simulink library "xps_library"  (R2018a)
settings: Solver=ode45  StartTime=0.0  StopTime=10.0  RelTol=1e-3
undefined symbols (not defined in the file or in its folder): ip_name, lib_path
libraries: xbsIndex_r4 x2454, casper_library_flow_control x68, simulink x52, $bdroot x22, casper_library_misc x9
(part 5 of 27)

== system xps_library/ADCs/rfdc_V0_1 ==
  ch0_sim_a : Inport
  sim_sync : Inport  Port=2
  sim_ad_clk : Inport  Port=3
  ch0_delay_a{0..7} (8 alike) : Delay  DelayLength=1  InitialCondition=0  InputProcessing=Inherited
  ch0_downsample_a0 : DownSample  N=8  RateOptions=Allow multirate processing
  ch0_downsample_a1 : DownSample  N=8  phase=1  RateOptions=Allow multirate processing
  ch0_downsample_a2 : DownSample  N=8  phase=2  RateOptions=Allow multirate processing
  ch0_downsample_a3 : DownSample  N=8  phase=3  RateOptions=Allow multirate processing
  ch0_downsample_a4 : DownSample  N=8  phase=4  RateOptions=Allow multirate processing
  ch0_downsample_a5 : DownSample  N=8  phase=5  RateOptions=Allow multirate processing
  ch0_downsample_a6 : DownSample  N=8  phase=6  RateOptions=Allow multirate processing
  ch0_downsample_a7 : DownSample  N=8  phase=7  RateOptions=Allow multirate processing
  xps_library_ADCs_rfdc_V0_1_adc0_clk : xbsIndex_r4/Gateway In  gui_display_data_type=Boolean  arith_type=Boolean  n_bits=16  bin_pt=14  preci_type=Single  exp_width=8  frac_width=24  rows=1  columns=1  quantization="Round  (unbiased: +/- Inf)"  overflow=Saturate  period=1  UseAsADC=off  ADCChannel='1'  interface=None  automatic_assignment=on  address_offset=hex2dec('00')  intf_name=''  intf_description=''  default_value=0  timing_constraint=None  locs_specified=off  LOCs={}  io_standard={}  inherit_from_input=off  hdl_port=on  dbl_ovrd=off  block_type=gatewayin
  xps_library_ADCs_rfdc_V0_1_adc0_dout_{0..7} (8 alike) : xbsIndex_r4/Gateway In  gui_display_data_type=Fixed-point  arith_type=Unsigned  n_bits=16  bin_pt=0  preci_type=Single  exp_width=8  frac_width=24  rows=1  columns=1  quantization=Truncate  overflow=Wrap  period=1  UseAsADC=off  ADCChannel='1'  interface=None  automatic_assignment=on  address_offset=hex2dec('00')  intf_name=''  intf_description=''  default_value=0  timing_constraint=None  locs_specified=off  LOCs={}  io_standard={}  inherit_from_input=off  hdl_port=on  dbl_ovrd=off  block_type=gatewayin
  xps_library_ADCs_rfdc_V0_1_adc0_sync : xbsIndex_r4/Gateway In  gui_display_data_type=Boolean  arith_type=Boolean  n_bits=16  bin_pt=14  preci_type=Single  exp_width=8  frac_width=24  rows=1  columns=1  quantization="Round  (unbiased: +/- Inf)"  overflow=Saturate  period=1  UseAsADC=off  ADCChannel='1'  interface=None  automatic_assignment=on  address_offset=hex2dec('00')  intf_name=''  intf_description=''  default_value=0  timing_constraint=None  locs_specified=off  LOCs={}  io_standard={}  inherit_from_input=off  hdl_port=on  dbl_ovrd=off  block_type=gatewayin
  ch0_a0 : Outport
  ch0_a1 : Outport  Port=2
  ch0_a2 : Outport  Port=3
  ch0_a3 : Outport  Port=4
  ch0_a4 : Outport  Port=5
  ch0_a5 : Outport  Port=6
  ch0_a6 : Outport  Port=7
  ch0_a7 : Outport  Port=8
  sync_out : Outport  Port=9
  ad_clk_out : Outport  Port=10
  wires:
  ch0_sim_a/1 -> ch0_downsample_a2/1, ch0_downsample_a1/1, ch0_downsample_a3/1, ch0_downsample_a0/1, ch0_downsample_a4/1, ch0_downsample_a5/1, ch0_downsample_a6/1, ch0_downsample_a7/1
  ch0_downsample_a4/1 -> ch0_delay_a4/1
  ch0_downsample_a5/1 -> ch0_delay_a5/1
  ch0_downsample_a7/1 -> ch0_delay_a7/1
  xps_library_ADCs_rfdc_V0_1_adc0_dout_5/1 -> ch0_a5/1
  xps_library_ADCs_rfdc_V0_1_adc0_dout_4/1 -> ch0_a4/1
  ch0_delay_a4/1 -> xps_library_ADCs_rfdc_V0_1_adc0_dout_4/1
  xps_library_ADCs_rfdc_V0_1_adc0_dout_6/1 -> ch0_a6/1
  ch0_delay_a6/1 -> xps_library_ADCs_rfdc_V0_1_adc0_dout_6/1
  ch0_delay_a7/1 -> xps_library_ADCs_rfdc_V0_1_adc0_dout_7/1
  xps_library_ADCs_rfdc_V0_1_adc0_dout_7/1 -> ch0_a7/1
  ch0_downsample_a6/1 -> ch0_delay_a6/1
  ch0_delay_a5/1 -> xps_library_ADCs_rfdc_V0_1_adc0_dout_5/1
  xps_library_ADCs_rfdc_V0_1_adc0_clk/1 -> ad_clk_out/1
  sim_ad_clk/1 -> xps_library_ADCs_rfdc_V0_1_adc0_clk/1
  xps_library_ADCs_rfdc_V0_1_adc0_sync/1 -> sync_out/1
  sim_sync/1 -> xps_library_ADCs_rfdc_V0_1_adc0_sync/1
  xps_library_ADCs_rfdc_V0_1_adc0_dout_3/1 -> ch0_a3/1
  ch0_delay_a3/1 -> xps_library_ADCs_rfdc_V0_1_adc0_dout_3/1
  ch0_downsample_a3/1 -> ch0_delay_a3/1
  xps_library_ADCs_rfdc_V0_1_adc0_dout_2/1 -> ch0_a2/1
  ch0_delay_a2/1 -> xps_library_ADCs_rfdc_V0_1_adc0_dout_2/1
  ch0_downsample_a2/1 -> ch0_delay_a2/1
  xps_library_ADCs_rfdc_V0_1_adc0_dout_1/1 -> ch0_a1/1
  ch0_delay_a1/1 -> xps_library_ADCs_rfdc_V0_1_adc0_dout_1/1
  ch0_downsample_a1/1 -> ch0_delay_a1/1
  xps_library_ADCs_rfdc_V0_1_adc0_dout_0/1 -> ch0_a0/1
  ch0_delay_a0/1 -> xps_library_ADCs_rfdc_V0_1_adc0_dout_0/1
  ch0_downsample_a0/1 -> ch0_delay_a0/1

== system xps_library/ADCs/rfdc_V0_2 ==
  adc0_in_sim : Inport
  adc0_sync_in_sim : Inport  Port=2
  dac0_din : Inport  Port=3
  dac0_valid_in : Inport  Port=4
  Terminator : Terminator
  Terminator1 : Terminator
  rfdc_V0_2_rfdc_V0_2_adc0_dout : xbsIndex_r4/Gateway In  gui_display_data_type=Fixed-point  arith_type=Unsigned  n_bits=128  bin_pt=0  preci_type=Single  exp_width=8  frac_width=24  rows=1  columns=1  quantization=Truncate  overflow=Wrap  period=1  UseAsADC=off  ADCChannel='1'  interface=None  automatic_assignment=on  address_offset=hex2dec('00')  intf_name=''  intf_description=''  default_value=0  timing_constraint=None  locs_specified=off  LOCs={}  io_standard={}  inherit_from_input=off  hdl_port=on  dbl_ovrd=off  block_type=gatewayin
  rfdc_V0_2_rfdc_V0_2_adc0_sync : xbsIndex_r4/Gateway In  gui_display_data_type=Fixed-point  arith_type=Boolean  n_bits=1  bin_pt=0  preci_type=Single  exp_width=8  frac_width=24  rows=1  columns=1  quantization=Truncate  overflow=Wrap  period=1  UseAsADC=off  ADCChannel='1'  interface=None  automatic_assignment=on  address_offset=hex2dec('00')  intf_name=''  intf_description=''  default_value=0  timing_constraint=None  locs_specified=off  LOCs={}  io_standard={}  inherit_from_input=off  hdl_port=on  dbl_ovrd=off  block_type=gatewayin
  rfdc_V0_2_rfdc_V0_2_dac0_din : xbsIndex_r4/Gateway Out  inherit_from_input=off  hdl_port=on  rows=1  columns=1  UseAsDAC=off  DACChannel='1'  interface=None  automatic_assignment=on  address_offset=hex2dec('00')  intf_name=''  intf_description=''  timing_constraint=None  locs_specified=off  LOCs={}  io_standard={}  block_type=gatewayout
  rfdc_V0_2_rfdc_V0_2_dac0_valid : xbsIndex_r4/Gateway Out  inherit_from_input=off  hdl_port=on  rows=1  columns=1  UseAsDAC=off  DACChannel='1'  interface=None  automatic_assignment=on  address_offset=hex2dec('00')  intf_name=''  intf_description=''  timing_constraint=None  locs_specified=off  LOCs={}  io_standard={}  block_type=gatewayout
  adc0_dout : Outport
  adc0_sync_out : Outport  Port=2
  wires:
  rfdc_V0_2_rfdc_V0_2_dac0_valid/1 -> Terminator1/1
  dac0_valid_in/1 -> rfdc_V0_2_rfdc_V0_2_dac0_valid/1
  rfdc_V0_2_rfdc_V0_2_dac0_din/1 -> Terminator/1
  dac0_din/1 -> rfdc_V0_2_rfdc_V0_2_dac0_din/1
  rfdc_V0_2_rfdc_V0_2_adc0_sync/1 -> adc0_sync_out/1
  adc0_sync_in_sim/1 -> rfdc_V0_2_rfdc_V0_2_adc0_sync/1
  rfdc_V0_2_rfdc_V0_2_adc0_dout/1 -> adc0_dout/1
  adc0_in_sim/1 -> rfdc_V0_2_rfdc_V0_2_adc0_dout/1

== system xps_library/ADCs/rfdc_V0_3 ==
  adc0_in_sim : Inport
  adc0_sync_in_sim : Inport  Port=2
  rfdc_V0_3_rfdc_V0_3_adc0_dout : xbsIndex_r4/Gateway In  gui_display_data_type=Fixed-point  arith_type=Unsigned  n_bits=128  bin_pt=0  preci_type=Single  exp_width=8  frac_width=24  rows=1  columns=1  quantization=Truncate  overflow=Wrap  period=1  UseAsADC=off  ADCChannel='1'  interface=None  automatic_assignment=on  address_offset=hex2dec('00')  intf_name=''  intf_description=''  default_value=0  timing_constraint=None  locs_specified=off  LOCs={}  io_standard={}  inherit_from_input=off  hdl_port=on  dbl_ovrd=off  block_type=gatewayin
  rfdc_V0_3_rfdc_V0_3_adc0_sync : xbsIndex_r4/Gateway In  gui_display_data_type=Fixed-point  arith_type=Boolean  n_bits=1  bin_pt=0  preci_type=Single  exp_width=8  frac_width=24  rows=1  columns=1  quantization=Truncate  overflow=Wrap  period=1  UseAsADC=off  ADCChannel='1'  interface=None  automatic_assignment=on  address_offset=hex2dec('00')  intf_name=''  intf_description=''  default_value=0  timing_constraint=None  locs_specified=off  LOCs={}  io_standard={}  inherit_from_input=off  hdl_port=on  dbl_ovrd=off  block_type=gatewayin
  adc0_dout : Outport
  adc0_sync_out : Outport  Port=2
  wires:
  rfdc_V0_3_rfdc_V0_3_adc0_sync/1 -> adc0_sync_out/1
  adc0_sync_in_sim/1 -> rfdc_V0_3_rfdc_V0_3_adc0_sync/1
  rfdc_V0_3_rfdc_V0_3_adc0_dout/1 -> adc0_dout/1
  adc0_in_sim/1 -> rfdc_V0_3_rfdc_V0_3_adc0_dout/1

== system xps_library/ADCs/rfdc_V0_4 ==
  adc0_in_sim : Inport
  adc0_sync_in_sim : Inport  Port=2
  rfdc_V0_4_rfdc_V0_4_adc0_dout : xbsIndex_r4/Gateway In  gui_display_data_type=Fixed-point  arith_type=Unsigned  n_bits=128  bin_pt=0  preci_type=Single  exp_width=8  frac_width=24  rows=1  columns=1  quantization=Truncate  overflow=Wrap  period=1  UseAsADC=off  ADCChannel='1'  interface=None  automatic_assignment=on  address_offset=hex2dec('00')  intf_name=''  intf_description=''  default_value=0  timing_constraint=None  locs_specified=off  LOCs={}  io_standard={}  inherit_from_input=off  hdl_port=on  dbl_ovrd=off  block_type=gatewayin
  rfdc_V0_4_rfdc_V0_4_adc0_sync : xbsIndex_r4/Gateway In  gui_display_data_type=Fixed-point  arith_type=Boolean  n_bits=1  bin_pt=0  preci_type=Single  exp_width=8  frac_width=24  rows=1  columns=1  quantization=Truncate  overflow=Wrap  period=1  UseAsADC=off  ADCChannel='1'  interface=None  automatic_assignment=on  address_offset=hex2dec('00')  intf_name=''  intf_description=''  default_value=0  timing_constraint=None  locs_specified=off  LOCs={}  io_standard={}  inherit_from_input=off  hdl_port=on  dbl_ovrd=off  block_type=gatewayin
  adc0_dout : Outport
  adc0_sync_out : Outport  Port=2
  wires:
  rfdc_V0_4_rfdc_V0_4_adc0_sync/1 -> adc0_sync_out/1
  adc0_sync_in_sim/1 -> rfdc_V0_4_rfdc_V0_4_adc0_sync/1
  rfdc_V0_4_rfdc_V0_4_adc0_dout/1 -> adc0_dout/1
  adc0_in_sim/1 -> rfdc_V0_4_rfdc_V0_4_adc0_dout/1

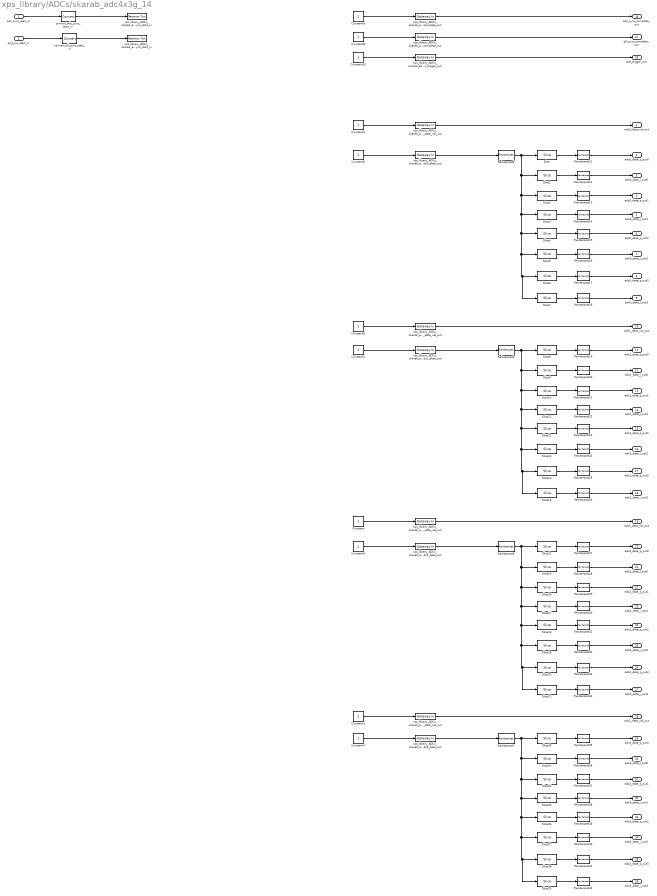
== system xps_library/ADCs/skarab_adc4x3g_14 ==
  adc_sync_start_in : Inport
  pll_sync_start_in : Inport  Port=2
  Constant{,1..10} (11 alike) : Constant
  Reinterpret{11..42} (32 alike) : xbsIndex_r4/Reinterpret  force_arith_type=on  arith_type="Signed  (2's comp)"  force_bin_pt=on  bin_pt=15  block_type=reinterpret
  Reinterpret{4..7} (4 alike) : xbsIndex_r4/Reinterpret  force_arith_type=on  arith_type=Unsigned  force_bin_pt=on  bin_pt=0  block_type=reinterpret
  Slice{,8,22,30} (4 alike) : xbsIndex_r4/Slice  nbits=16  boolean_output=off  mode=Lower Bit Location + Width  bit1=0  base1=MSB of Input  bit0=0  base0=LSB of Input  dbl_ovrd=off  block_type=slice
  Slice{1,9,23,31} (4 alike) : xbsIndex_r4/Slice  nbits=16  boolean_output=off  mode=Lower Bit Location + Width  bit1=0  base1=MSB of Input  bit0=16  base0=LSB of Input  dbl_ovrd=off  block_type=slice
  Slice{2,10,16,24} (4 alike) : xbsIndex_r4/Slice  nbits=16  boolean_output=off  mode=Lower Bit Location + Width  bit1=0  base1=MSB of Input  bit0=32  base0=LSB of Input  dbl_ovrd=off  block_type=slice
  Slice{3,11,17,25} (4 alike) : xbsIndex_r4/Slice  nbits=16  boolean_output=off  mode=Lower Bit Location + Width  bit1=0  base1=MSB of Input  bit0=48  base0=LSB of Input  dbl_ovrd=off  block_type=slice
  Slice{4,12,18,26} (4 alike) : xbsIndex_r4/Slice  nbits=16  boolean_output=off  mode=Lower Bit Location + Width  bit1=0  base1=MSB of Input  bit0=64  base0=LSB of Input  dbl_ovrd=off  block_type=slice
  Slice{5,13,19,27} (4 alike) : xbsIndex_r4/Slice  nbits=16  boolean_output=off  mode=Lower Bit Location + Width  bit1=0  base1=MSB of Input  bit0=80  base0=LSB of Input  dbl_ovrd=off  block_type=slice
  Slice{6,14,20,28} (4 alike) : xbsIndex_r4/Slice  nbits=16  boolean_output=off  mode=Lower Bit Location + Width  bit1=0  base1=MSB of Input  bit0=96  base0=LSB of Input  dbl_ovrd=off  block_type=slice
  Slice{7,15,21,29} (4 alike) : xbsIndex_r4/Slice  nbits=16  boolean_output=off  mode=Lower Bit Location + Width  bit1=0  base1=MSB of Input  bit0=112  base0=LSB of Input  dbl_ovrd=off  block_type=slice
  convert_adc_sync_start_in : xbsIndex_r4/Convert  gui_display_data_type=Boolean  arith_type=Boolean  n_bits=16  bin_pt=14  float_type=Single  exp_bits=8  fraction_bits=24  quantization=Truncate  overflow=Wrap  en=off  latency=0  pipeline=off  dbl_ovrd=off  block_type=convert
  convert_pll_sync_start_in : xbsIndex_r4/Convert  gui_display_data_type=Boolean  arith_type=Boolean  n_bits=16  bin_pt=14  float_type=Single  exp_bits=8  fraction_bits=24  quantization=Truncate  overflow=Wrap  en=off  latency=0  pipeline=off  dbl_ovrd=off  block_type=convert
  xps_library_ADCs_skarab_adc4x3g_14_adc0_data_out : xbsIndex_r4/Gateway In  gui_display_data_type=Fixed-point  arith_type=Unsigned  n_bits=128  bin_pt=0  preci_type=Single  exp_width=8  frac_width=24  rows=1  columns=1  quantization=Truncate  overflow=Wrap  period=1  UseAsADC=off  ADCChannel='1'  interface=None  automatic_assignment=on  address_offset=hex2dec('00')  intf_name=''  intf_description=''  default_value=0  timing_constraint=None  locs_specified=off  LOCs={}  io_standard={}  inherit_from_input=off  hdl_port=on  dbl_ovrd=off  block_type=gatewayin
  xps_library_ADCs_skarab_adc4x3g_14_adc0_data_val_out : xbsIndex_r4/Gateway In  gui_display_data_type=Boolean  arith_type=Boolean  n_bits=16  bin_pt=14  preci_type=Single  exp_width=8  frac_width=24  rows=1  columns=1  quantization="Round  (unbiased: +/- Inf)"  overflow=Saturate  period=1  UseAsADC=off  ADCChannel='1'  interface=None  automatic_assignment=on  address_offset=hex2dec('00')  intf_name=''  intf_description=''  default_value=0  timing_constraint=None  locs_specified=off  LOCs={}  io_standard={}  inherit_from_input=off  hdl_port=on  dbl_ovrd=off  block_type=gatewayin
  xps_library_ADCs_skarab_adc4x3g_14_adc1_data_out : xbsIndex_r4/Gateway In  gui_display_data_type=Fixed-point  arith_type=Unsigned  n_bits=128  bin_pt=0  preci_type=Single  exp_width=8  frac_width=24  rows=1  columns=1  quantization=Truncate  overflow=Wrap  period=1  UseAsADC=off  ADCChannel='1'  interface=None  automatic_assignment=on  address_offset=hex2dec('00')  intf_name=''  intf_description=''  default_value=0  timing_constraint=None  locs_specified=off  LOCs={}  io_standard={}  inherit_from_input=off  hdl_port=on  dbl_ovrd=off  block_type=gatewayin
  xps_library_ADCs_skarab_adc4x3g_14_adc1_data_val_out : xbsIndex_r4/Gateway In  gui_display_data_type=Boolean  arith_type=Boolean  n_bits=16  bin_pt=14  preci_type=Single  exp_width=8  frac_width=24  rows=1  columns=1  quantization="Round  (unbiased: +/- Inf)"  overflow=Saturate  period=1  UseAsADC=off  ADCChannel='1'  interface=None  automatic_assignment=on  address_offset=hex2dec('00')  intf_name=''  intf_description=''  default_value=0  timing_constraint=None  locs_specified=off  LOCs={}  io_standard={}  inherit_from_input=off  hdl_port=on  dbl_ovrd=off  block_type=gatewayin
  xps_library_ADCs_skarab_adc4x3g_14_adc2_data_out : xbsIndex_r4/Gateway In  gui_display_data_type=Fixed-point  arith_type=Unsigned  n_bits=128  bin_pt=0  preci_type=Single  exp_width=8  frac_width=24  rows=1  columns=1  quantization=Truncate  overflow=Wrap  period=1  UseAsADC=off  ADCChannel='1'  interface=None  automatic_assignment=on  address_offset=hex2dec('00')  intf_name=''  intf_description=''  default_value=0  timing_constraint=None  locs_specified=off  LOCs={}  io_standard={}  inherit_from_input=off  hdl_port=on  dbl_ovrd=off  block_type=gatewayin
  xps_library_ADCs_skarab_adc4x3g_14_adc2_data_val_out : xbsIndex_r4/Gateway In  gui_display_data_type=Boolean  arith_type=Boolean  n_bits=16  bin_pt=14  preci_type=Single  exp_width=8  frac_width=24  rows=1  columns=1  quantization="Round  (unbiased: +/- Inf)"  overflow=Saturate  period=1  UseAsADC=off  ADCChannel='1'  interface=None  automatic_assignment=on  address_offset=hex2dec('00')  intf_name=''  intf_description=''  default_value=0  timing_constraint=None  locs_specified=off  LOCs={}  io_standard={}  inherit_from_input=off  hdl_port=on  dbl_ovrd=off  block_type=gatewayin
  xps_library_ADCs_skarab_adc4x3g_14_adc3_data_out : xbsIndex_r4/Gateway In  gui_display_data_type=Fixed-point  arith_type=Unsigned  n_bits=128  bin_pt=0  preci_type=Single  exp_width=8  frac_width=24  rows=1  columns=1  quantization=Truncate  overflow=Wrap  period=1  UseAsADC=off  ADCChannel='1'  interface=None  automatic_assignment=on  address_offset=hex2dec('00')  intf_name=''  intf_description=''  default_value=0  timing_constraint=None  locs_specified=off  LOCs={}  io_standard={}  inherit_from_input=off  hdl_port=on  dbl_ovrd=off  block_type=gatewayin
  xps_library_ADCs_skarab_adc4x3g_14_adc3_data_val_out : xbsIndex_r4/Gateway In  gui_display_data_type=Boolean  arith_type=Boolean  n_bits=16  bin_pt=14  preci_type=Single  exp_width=8  frac_width=24  rows=1  columns=1  quantization="Round  (unbiased: +/- Inf)"  overflow=Saturate  period=1  UseAsADC=off  ADCChannel='1'  interface=None  automatic_assignment=on  address_offset=hex2dec('00')  intf_name=''  intf_description=''  default_value=0  timing_constraint=None  locs_specified=off  LOCs={}  io_standard={}  inherit_from_input=off  hdl_port=on  dbl_ovrd=off  block_type=gatewayin
  xps_library_ADCs_skarab_adc4x3g_14_adc_sync_complete_out : xbsIndex_r4/Gateway In  gui_display_data_type=Boolean  arith_type=Boolean  n_bits=16  bin_pt=14  preci_type=Single  exp_width=8  frac_width=24  rows=1  columns=1  quantization="Round  (unbiased: +/- Inf)"  overflow=Saturate  period=1  UseAsADC=off  ADCChannel='1'  interface=None  automatic_assignment=on  address_offset=hex2dec('00')  intf_name=''  intf_description=''  default_value=0  timing_constraint=None  locs_specified=off  LOCs={}  io_standard={}  inherit_from_input=off  hdl_port=on  dbl_ovrd=off  block_type=gatewayin
  xps_library_ADCs_skarab_adc4x3g_14_adc_sync_start_in : xbsIndex_r4/Gateway Out  inherit_from_input=off  hdl_port=on  rows=1  columns=1  UseAsDAC=off  DACChannel='1'  interface=None  automatic_assignment=on  address_offset=hex2dec('00')  intf_name=''  intf_description=''  timing_constraint=None  locs_specified=off  LOCs={}  io_standard={}  block_type=gatewayout
  xps_library_ADCs_skarab_adc4x3g_14_adc_trigger_out : xbsIndex_r4/Gateway In  gui_display_data_type=Boolean  arith_type=Boolean  n_bits=16  bin_pt=14  preci_type=Single  exp_width=8  frac_width=24  rows=1  columns=1  quantization="Round  (unbiased: +/- Inf)"  overflow=Saturate  period=1  UseAsADC=off  ADCChannel='1'  interface=None  automatic_assignment=on  address_offset=hex2dec('00')  intf_name=''  intf_description=''  default_value=0  timing_constraint=None  locs_specified=off  LOCs={}  io_standard={}  inherit_from_input=off  hdl_port=on  dbl_ovrd=off  block_type=gatewayin
  xps_library_ADCs_skarab_adc4x3g_14_pll_sync_complete_out : xbsIndex_r4/Gateway In  gui_display_data_type=Boolean  arith_type=Boolean  n_bits=16  bin_pt=14  preci_type=Single  exp_width=8  frac_width=24  rows=1  columns=1  quantization="Round  (unbiased: +/- Inf)"  overflow=Saturate  period=1  UseAsADC=off  ADCChannel='1'  interface=None  automatic_assignment=on  address_offset=hex2dec('00')  intf_name=''  intf_description=''  default_value=0  timing_constraint=None  locs_specified=off  LOCs={}  io_standard={}  inherit_from_input=off  hdl_port=on  dbl_ovrd=off  block_type=gatewayin
  xps_library_ADCs_skarab_adc4x3g_14_pll_sync_start_in : xbsIndex_r4/Gateway Out  inherit_from_input=off  hdl_port=on  rows=1  columns=1  UseAsDAC=off  DACChannel='1'  interface=None  automatic_assignment=on  address_offset=hex2dec('00')  intf_name=''  intf_description=''  timing_constraint=None  locs_specified=off  LOCs={}  io_standard={}  block_type=gatewayout
  adc0_data_val_out : Outport
  adc0_data_q_out0 : Outport  Port=2
  adc0_data_i_out0 : Outport  Port=3
  adc0_data_q_out1 : Outport  Port=4
  adc0_data_i_out1 : Outport  Port=5
  adc0_data_q_out2 : Outport  Port=6
  adc0_data_i_out2 : Outport  Port=7
  adc0_data_q_out3 : Outport  Port=8
  adc0_data_i_out3 : Outport  Port=9
  adc1_data_val_out : Outport  Port=10
  adc1_data_q_out0 : Outport  Port=11
  adc1_data_i_out0 : Outport  Port=12
  adc1_data_q_out1 : Outport  Port=13
  adc1_data_i_out1 : Outport  Port=14
  adc1_data_q_out2 : Outport  Port=15
  adc1_data_i_out2 : Outport  Port=16
  adc1_data_q_out3 : Outport  Port=17
  adc1_data_i_out3 : Outport  Port=18
  adc2_data_val_out : Outport  Port=19
  adc2_data_q_out0 : Outport  Port=20
  adc2_data_i_out0 : Outport  Port=21
  adc2_data_q_out1 : Outport  Port=22
  adc2_data_i_out1 : Outport  Port=23
  adc2_data_q_out2 : Outport  Port=24
  adc2_data_i_out2 : Outport  Port=25
  adc2_data_q_out3 : Outport  Port=26
  adc2_data_i_out3 : Outport  Port=27
  adc3_data_val_out : Outport  Port=28
  adc3_data_q_out0 : Outport  Port=29
  adc3_data_i_out0 : Outport  Port=30
  adc3_data_q_out1 : Outport  Port=31
  adc3_data_i_out1 : Outport  Port=32
  adc3_data_q_out2 : Outport  Port=33
  adc3_data_i_out2 : Outport  Port=34
  adc3_data_q_out3 : Outport  Port=35
  adc3_data_i_out3 : Outport  Port=36
  pll_sync_complete_out : Outport  Port=37
  adc_sync_complete_out : Outport  Port=38
  adc_trigger_out : Outport  Port=39
  wires:
  xps_library_ADCs_skarab_adc4x3g_14_adc_trigger_out/1 -> adc_trigger_out/1
  Constant10/1 -> xps_library_ADCs_skarab_adc4x3g_14_adc_trigger_out/1
  xps_library_ADCs_skarab_adc4x3g_14_adc_sync_complete_out/1 -> adc_sync_complete_out/1
  Constant9/1 -> xps_library_ADCs_skarab_adc4x3g_14_adc_sync_complete_out/1
  xps_library_ADCs_skarab_adc4x3g_14_pll_sync_complete_out/1 -> pll_sync_complete_out/1
  Constant8/1 -> xps_library_ADCs_skarab_adc4x3g_14_pll_sync_complete_out/1
  Slice29/1 -> Reinterpret42/1
  Reinterpret42/1 -> adc3_data_i_out3/1
  Slice28/1 -> Reinterpret41/1
  Reinterpret41/1 -> adc3_data_q_out3/1
  Slice27/1 -> Reinterpret40/1
  Reinterpret40/1 -> adc3_data_i_out2/1
  Slice26/1 -> Reinterpret39/1
  Reinterpret39/1 -> adc3_data_q_out2/1
  Slice25/1 -> Reinterpret38/1
  Reinterpret38/1 -> adc3_data_i_out1/1
  Slice24/1 -> Reinterpret37/1
  Reinterpret37/1 -> adc3_data_q_out1/1
  Slice31/1 -> Reinterpret36/1
  Reinterpret36/1 -> adc3_data_i_out0/1
  Slice30/1 -> Reinterpret35/1
  Reinterpret35/1 -> adc3_data_q_out0/1
  Reinterpret7/1 -> Slice30/1, Slice31/1, Slice24/1, Slice25/1, Slice26/1, Slice27/1, Slice28/1, Slice29/1
  xps_library_ADCs_skarab_adc4x3g_14_adc3_data_out/1 -> Reinterpret7/1
  Constant7/1 -> xps_library_ADCs_skarab_adc4x3g_14_adc3_data_out/1
  Slice21/1 -> Reinterpret34/1
  Reinterpret34/1 -> adc2_data_i_out3/1
  Slice20/1 -> Reinterpret33/1
  Reinterpret33/1 -> adc2_data_q_out3/1
  Slice19/1 -> Reinterpret32/1
  Reinterpret32/1 -> adc2_data_i_out2/1
  Slice18/1 -> Reinterpret31/1
  Reinterpret31/1 -> adc2_data_q_out2/1
  Slice17/1 -> Reinterpret30/1
  Reinterpret30/1 -> adc2_data_i_out1/1
  Slice16/1 -> Reinterpret29/1
  Reinterpret29/1 -> adc2_data_q_out1/1
  Slice23/1 -> Reinterpret28/1
  Reinterpret28/1 -> adc2_data_i_out0/1
  Slice22/1 -> Reinterpret27/1
  Reinterpret27/1 -> adc2_data_q_out0/1
  Reinterpret5/1 -> Slice22/1, Slice23/1, Slice16/1, Slice17/1, Slice18/1, Slice19/1, Slice20/1, Slice21/1
  xps_library_ADCs_skarab_adc4x3g_14_adc2_data_out/1 -> Reinterpret5/1
  Constant3/1 -> xps_library_ADCs_skarab_adc4x3g_14_adc2_data_out/1
  Slice15/1 -> Reinterpret26/1
  Reinterpret26/1 -> adc1_data_i_out3/1
  Slice14/1 -> Reinterpret25/1
  Reinterpret25/1 -> adc1_data_q_out3/1
  Slice13/1 -> Reinterpret24/1
  Reinterpret24/1 -> adc1_data_i_out2/1
  Slice12/1 -> Reinterpret23/1
  Reinterpret23/1 -> adc1_data_q_out2/1
  Slice11/1 -> Reinterpret22/1
  Reinterpret22/1 -> adc1_data_i_out1/1
  Slice10/1 -> Reinterpret21/1
  Reinterpret21/1 -> adc1_data_q_out1/1
  Slice9/1 -> Reinterpret20/1
  Reinterpret20/1 -> adc1_data_i_out0/1
  Slice8/1 -> Reinterpret19/1
  Reinterpret19/1 -> adc1_data_q_out0/1
  Reinterpret4/1 -> Slice8/1, Slice9/1, Slice10/1, Slice11/1, Slice12/1, Slice13/1, Slice14/1, Slice15/1
  xps_library_ADCs_skarab_adc4x3g_14_adc1_data_out/1 -> Reinterpret4/1
  Constant2/1 -> xps_library_ADCs_skarab_adc4x3g_14_adc1_data_out/1
  Slice7/1 -> Reinterpret18/1
  Reinterpret18/1 -> adc0_data_i_out3/1
  Slice6/1 -> Reinterpret17/1
  Reinterpret17/1 -> adc0_data_q_out3/1
  Slice5/1 -> Reinterpret16/1
  Reinterpret16/1 -> adc0_data_i_out2/1
  Slice4/1 -> Reinterpret15/1
  Reinterpret15/1 -> adc0_data_q_out2/1
  Slice3/1 -> Reinterpret14/1
  Reinterpret14/1 -> adc0_data_i_out1/1
  Slice2/1 -> Reinterpret13/1
  Reinterpret13/1 -> adc0_data_q_out1/1
  Slice1/1 -> Reinterpret12/1
  Reinterpret12/1 -> adc0_data_i_out0/1
  Slice/1 -> Reinterpret11/1
  Reinterpret11/1 -> adc0_data_q_out0/1
  Reinterpret6/1 -> Slice/1, Slice1/1, Slice2/1, Slice3/1, Slice4/1, Slice5/1, Slice6/1, Slice7/1
  xps_library_ADCs_skarab_adc4x3g_14_adc0_data_out/1 -> Reinterpret6/1
  Constant6/1 -> xps_library_ADCs_skarab_adc4x3g_14_adc0_data_out/1
  xps_library_ADCs_skarab_adc4x3g_14_adc1_data_val_out/1 -> adc1_data_val_out/1
  Constant5/1 -> xps_library_ADCs_skarab_adc4x3g_14_adc1_data_val_out/1
  xps_library_ADCs_skarab_adc4x3g_14_adc0_data_val_out/1 -> adc0_data_val_out/1
  Constant4/1 -> xps_library_ADCs_skarab_adc4x3g_14_adc0_data_val_out/1
  xps_library_ADCs_skarab_adc4x3g_14_adc3_data_val_out/1 -> adc3_data_val_out/1
  Constant1/1 -> xps_library_ADCs_skarab_adc4x3g_14_adc3_data_val_out/1
  xps_library_ADCs_skarab_adc4x3g_14_adc2_data_val_out/1 -> adc2_data_val_out/1
  Constant/1 -> xps_library_ADCs_skarab_adc4x3g_14_adc2_data_val_out/1
  convert_pll_sync_start_in/1 -> xps_library_ADCs_skarab_adc4x3g_14_pll_sync_start_in/1
  pll_sync_start_in/1 -> convert_pll_sync_start_in/1
  convert_adc_sync_start_in/1 -> xps_library_ADCs_skarab_adc4x3g_14_adc_sync_start_in/1
  adc_sync_start_in/1 -> convert_adc_sync_start_in/1

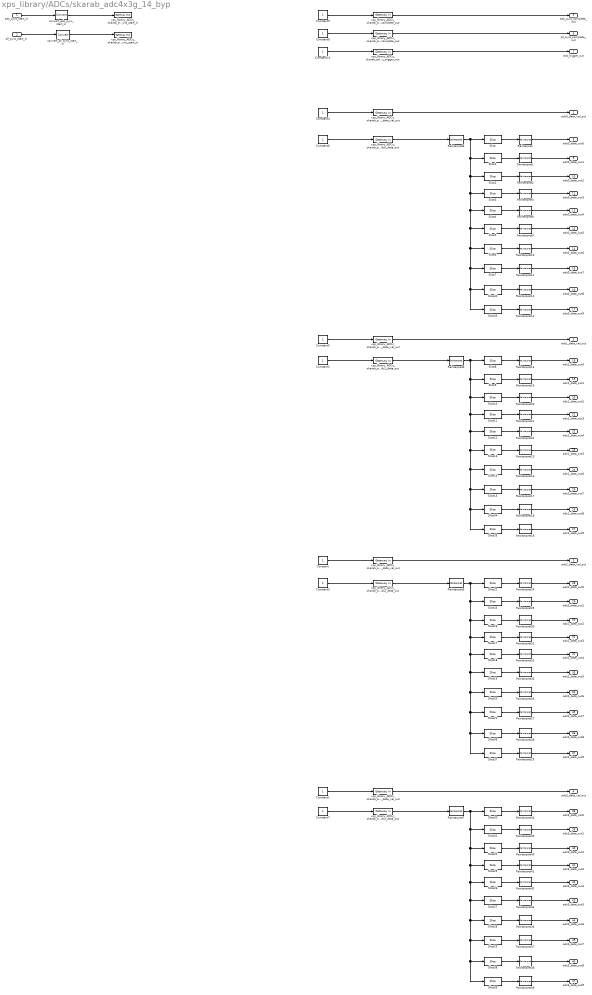
== system xps_library/ADCs/skarab_adc4x3g_14_byp ==
  adc_sync_start_in : Inport
  pll_sync_start_in : Inport  Port=2
  Constant{,1..10} (11 alike) : Constant
  Reinterpret{,1..3,8..43} (40 alike) : xbsIndex_r4/Reinterpret  force_arith_type=on  arith_type="Signed  (2's comp)"  force_bin_pt=on  bin_pt=11  block_type=reinterpret
  Reinterpret{4..7} (4 alike) : xbsIndex_r4/Reinterpret  force_arith_type=on  arith_type=Unsigned  force_bin_pt=on  bin_pt=0  block_type=reinterpret
  Slice{,8,22,30} (4 alike) : xbsIndex_r4/Slice  nbits=12  boolean_output=off  mode=Lower Bit Location + Width  bit1=0  base1=MSB of Input  bit0=0  base0=LSB of Input  dbl_ovrd=off  block_type=slice
  Slice{1,9,23,31} (4 alike) : xbsIndex_r4/Slice  nbits=12  boolean_output=off  mode=Lower Bit Location + Width  bit1=0  base1=MSB of Input  bit0=12  base0=LSB of Input  dbl_ovrd=off  block_type=slice
  Slice{2,10,16,24} (4 alike) : xbsIndex_r4/Slice  nbits=12  boolean_output=off  mode=Lower Bit Location + Width  bit1=0  base1=MSB of Input  bit0=24  base0=LSB of Input  dbl_ovrd=off  block_type=slice
  Slice{3,11,17,25} (4 alike) : xbsIndex_r4/Slice  nbits=12  boolean_output=off  mode=Lower Bit Location + Width  bit1=0  base1=MSB of Input  bit0=36  base0=LSB of Input  dbl_ovrd=off  block_type=slice
  Slice{4,12,18,26} (4 alike) : xbsIndex_r4/Slice  nbits=12  boolean_output=off  mode=Lower Bit Location + Width  bit1=0  base1=MSB of Input  bit0=48  base0=LSB of Input  dbl_ovrd=off  block_type=slice
  Slice{5,13,19,27} (4 alike) : xbsIndex_r4/Slice  nbits=12  boolean_output=off  mode=Lower Bit Location + Width  bit1=0  base1=MSB of Input  bit0=60  base0=LSB of Input  dbl_ovrd=off  block_type=slice
  Slice{6,14,20,28} (4 alike) : xbsIndex_r4/Slice  nbits=12  boolean_output=off  mode=Lower Bit Location + Width  bit1=0  base1=MSB of Input  bit0=72  base0=LSB of Input  dbl_ovrd=off  block_type=slice
  Slice{7,15,21,29} (4 alike) : xbsIndex_r4/Slice  nbits=12  boolean_output=off  mode=Lower Bit Location + Width  bit1=0  base1=MSB of Input  bit0=84  base0=LSB of Input  dbl_ovrd=off  block_type=slice
  Slice{32,34,36,38} (4 alike) : xbsIndex_r4/Slice  nbits=12  boolean_output=off  mode=Lower Bit Location + Width  bit1=0  base1=MSB of Input  bit0=96  base0=LSB of Input  dbl_ovrd=off  block_type=slice
  Slice{33,35,37,39} (4 alike) : xbsIndex_r4/Slice  nbits=12  boolean_output=off  mode=Lower Bit Location + Width  bit1=0  base1=MSB of Input  bit0=108  base0=LSB of Input  dbl_ovrd=off  block_type=slice
  convert_adc_sync_start_in : xbsIndex_r4/Convert  gui_display_data_type=Boolean  arith_type=Boolean  n_bits=16  bin_pt=14  float_type=Single  exp_bits=8  fraction_bits=24  quantization=Truncate  overflow=Wrap  en=off  latency=0  pipeline=off  dbl_ovrd=off  block_type=convert
  convert_pll_sync_start_in : xbsIndex_r4/Convert  gui_display_data_type=Boolean  arith_type=Boolean  n_bits=16  bin_pt=14  float_type=Single  exp_bits=8  fraction_bits=24  quantization=Truncate  overflow=Wrap  en=off  latency=0  pipeline=off  dbl_ovrd=off  block_type=convert
  xps_library_ADCs_skarab_adc4x3g_14_byp_adc0_data_out : xbsIndex_r4/Gateway In  gui_display_data_type=Fixed-point  arith_type=Unsigned  n_bits=128  bin_pt=0  preci_type=Single  exp_width=8  frac_width=24  rows=1  columns=1  quantization=Truncate  overflow=Wrap  period=1  UseAsADC=off  ADCChannel='1'  interface=None  automatic_assignment=on  address_offset=hex2dec('00')  intf_name=''  intf_description=''  default_value=0  timing_constraint=None  locs_specified=off  LOCs={}  io_standard={}  inherit_from_input=off  hdl_port=on  dbl_ovrd=off  block_type=gatewayin
  xps_library_ADCs_skarab_adc4x3g_14_byp_adc0_data_val_out : xbsIndex_r4/Gateway In  gui_display_data_type=Boolean  arith_type=Boolean  n_bits=16  bin_pt=14  preci_type=Single  exp_width=8  frac_width=24  rows=1  columns=1  quantization="Round  (unbiased: +/- Inf)"  overflow=Saturate  period=1  UseAsADC=off  ADCChannel='1'  interface=None  automatic_assignment=on  address_offset=hex2dec('00')  intf_name=''  intf_description=''  default_value=0  timing_constraint=None  locs_specified=off  LOCs={}  io_standard={}  inherit_from_input=off  hdl_port=on  dbl_ovrd=off  block_type=gatewayin
  xps_library_ADCs_skarab_adc4x3g_14_byp_adc1_data_out : xbsIndex_r4/Gateway In  gui_display_data_type=Fixed-point  arith_type=Unsigned  n_bits=128  bin_pt=0  preci_type=Single  exp_width=8  frac_width=24  rows=1  columns=1  quantization=Truncate  overflow=Wrap  period=1  UseAsADC=off  ADCChannel='1'  interface=None  automatic_assignment=on  address_offset=hex2dec('00')  intf_name=''  intf_description=''  default_value=0  timing_constraint=None  locs_specified=off  LOCs={}  io_standard={}  inherit_from_input=off  hdl_port=on  dbl_ovrd=off  block_type=gatewayin
  xps_library_ADCs_skarab_adc4x3g_14_byp_adc1_data_val_out : xbsIndex_r4/Gateway In  gui_display_data_type=Boolean  arith_type=Boolean  n_bits=16  bin_pt=14  preci_type=Single  exp_width=8  frac_width=24  rows=1  columns=1  quantization="Round  (unbiased: +/- Inf)"  overflow=Saturate  period=1  UseAsADC=off  ADCChannel='1'  interface=None  automatic_assignment=on  address_offset=hex2dec('00')  intf_name=''  intf_description=''  default_value=0  timing_constraint=None  locs_specified=off  LOCs={}  io_standard={}  inherit_from_input=off  hdl_port=on  dbl_ovrd=off  block_type=gatewayin
  xps_library_ADCs_skarab_adc4x3g_14_byp_adc2_data_out : xbsIndex_r4/Gateway In  gui_display_data_type=Fixed-point  arith_type=Unsigned  n_bits=128  bin_pt=0  preci_type=Single  exp_width=8  frac_width=24  rows=1  columns=1  quantization=Truncate  overflow=Wrap  period=1  UseAsADC=off  ADCChannel='1'  interface=None  automatic_assignment=on  address_offset=hex2dec('00')  intf_name=''  intf_description=''  default_value=0  timing_constraint=None  locs_specified=off  LOCs={}  io_standard={}  inherit_from_input=off  hdl_port=on  dbl_ovrd=off  block_type=gatewayin
  xps_library_ADCs_skarab_adc4x3g_14_byp_adc2_data_val_out : xbsIndex_r4/Gateway In  gui_display_data_type=Boolean  arith_type=Boolean  n_bits=16  bin_pt=14  preci_type=Single  exp_width=8  frac_width=24  rows=1  columns=1  quantization="Round  (unbiased: +/- Inf)"  overflow=Saturate  period=1  UseAsADC=off  ADCChannel='1'  interface=None  automatic_assignment=on  address_offset=hex2dec('00')  intf_name=''  intf_description=''  default_value=0  timing_constraint=None  locs_specified=off  LOCs={}  io_standard={}  inherit_from_input=off  hdl_port=on  dbl_ovrd=off  block_type=gatewayin
  xps_library_ADCs_skarab_adc4x3g_14_byp_adc3_data_out : xbsIndex_r4/Gateway In  gui_display_data_type=Fixed-point  arith_type=Unsigned  n_bits=128  bin_pt=0  preci_type=Single  exp_width=8  frac_width=24  rows=1  columns=1  quantization=Truncate  overflow=Wrap  period=1  UseAsADC=off  ADCChannel='1'  interface=None  automatic_assignment=on  address_offset=hex2dec('00')  intf_name=''  intf_description=''  default_value=0  timing_constraint=None  locs_specified=off  LOCs={}  io_standard={}  inherit_from_input=off  hdl_port=on  dbl_ovrd=off  block_type=gatewayin
  xps_library_ADCs_skarab_adc4x3g_14_byp_adc3_data_val_out : xbsIndex_r4/Gateway In  gui_display_data_type=Boolean  arith_type=Boolean  n_bits=16  bin_pt=14  preci_type=Single  exp_width=8  frac_width=24  rows=1  columns=1  quantization="Round  (unbiased: +/- Inf)"  overflow=Saturate  period=1  UseAsADC=off  ADCChannel='1'  interface=None  automatic_assignment=on  address_offset=hex2dec('00')  intf_name=''  intf_description=''  default_value=0  timing_constraint=None  locs_specified=off  LOCs={}  io_standard={}  inherit_from_input=off  hdl_port=on  dbl_ovrd=off  block_type=gatewayin
  xps_library_ADCs_skarab_adc4x3g_14_byp_adc_sync_complete_out : xbsIndex_r4/Gateway In  gui_display_data_type=Boolean  arith_type=Boolean  n_bits=16  bin_pt=14  preci_type=Single  exp_width=8  frac_width=24  rows=1  columns=1  quantization="Round  (unbiased: +/- Inf)"  overflow=Saturate  period=1  UseAsADC=off  ADCChannel='1'  interface=None  automatic_assignment=on  address_offset=hex2dec('00')  intf_name=''  intf_description=''  default_value=0  timing_constraint=None  locs_specified=off  LOCs={}  io_standard={}  inherit_from_input=off  hdl_port=on  dbl_ovrd=off  block_type=gatewayin
  xps_library_ADCs_skarab_adc4x3g_14_byp_adc_sync_start_in : xbsIndex_r4/Gateway Out  inherit_from_input=off  hdl_port=on  rows=1  columns=1  UseAsDAC=off  DACChannel='1'  interface=None  automatic_assignment=on  address_offset=hex2dec('00')  intf_name=''  intf_description=''  timing_constraint=None  locs_specified=off  LOCs={}  io_standard={}  block_type=gatewayout
  xps_library_ADCs_skarab_adc4x3g_14_byp_adc_trigger_out : xbsIndex_r4/Gateway In  gui_display_data_type=Boolean  arith_type=Boolean  n_bits=16  bin_pt=14  preci_type=Single  exp_width=8  frac_width=24  rows=1  columns=1  quantization="Round  (unbiased: +/- Inf)"  overflow=Saturate  period=1  UseAsADC=off  ADCChannel='1'  interface=None  automatic_assignment=on  address_offset=hex2dec('00')  intf_name=''  intf_description=''  default_value=0  timing_constraint=None  locs_specified=off  LOCs={}  io_standard={}  inherit_from_input=off  hdl_port=on  dbl_ovrd=off  block_type=gatewayin
  xps_library_ADCs_skarab_adc4x3g_14_byp_pll_sync_complete_out : xbsIndex_r4/Gateway In  gui_display_data_type=Boolean  arith_type=Boolean  n_bits=16  bin_pt=14  preci_type=Single  exp_width=8  frac_width=24  rows=1  columns=1  quantization="Round  (unbiased: +/- Inf)"  overflow=Saturate  period=1  UseAsADC=off  ADCChannel='1'  interface=None  automatic_assignment=on  address_offset=hex2dec('00')  intf_name=''  intf_description=''  default_value=0  timing_constraint=None  locs_specified=off  LOCs={}  io_standard={}  inherit_from_input=off  hdl_port=on  dbl_ovrd=off  block_type=gatewayin
  xps_library_ADCs_skarab_adc4x3g_14_byp_pll_sync_start_in : xbsIndex_r4/Gateway Out  inherit_from_input=off  hdl_port=on  rows=1  columns=1  UseAsDAC=off  DACChannel='1'  interface=None  automatic_assignment=on  address_offset=hex2dec('00')  intf_name=''  intf_description=''  timing_constraint=None  locs_specified=off  LOCs={}  io_standard={}  block_type=gatewayout
  adc0_data_val_out : Outport
  adc1_data_val_out : Outport  Port=2
  adc2_data_val_out : Outport  Port=3
  adc3_data_val_out : Outport  Port=4
  pll_sync_complete_out : Outport  Port=5
  adc_sync_complete_out : Outport  Port=6
  adc_trigger_out : Outport  Port=7
  adc0_data_out0 : Outport  Port=8
  adc0_data_out1 : Outport  Port=9
  adc0_data_out2 : Outport  Port=10
  adc0_data_out3 : Outport  Port=11
  adc0_data_out4 : Outport  Port=12
  adc0_data_out5 : Outport  Port=13
  adc0_data_out6 : Outport  Port=14
  adc0_data_out7 : Outport  Port=15
  adc0_data_out8 : Outport  Port=16
  adc0_data_out9 : Outport  Port=17
  adc1_data_out0 : Outport  Port=18
  adc1_data_out1 : Outport  Port=19
  adc1_data_out2 : Outport  Port=20
  adc1_data_out3 : Outport  Port=21
  adc1_data_out4 : Outport  Port=22
  adc1_data_out5 : Outport  Port=23
  adc1_data_out6 : Outport  Port=24
  adc1_data_out7 : Outport  Port=25
  adc1_data_out8 : Outport  Port=26
  adc1_data_out9 : Outport  Port=27
  adc2_data_out0 : Outport  Port=28
  adc2_data_out1 : Outport  Port=29
  adc2_data_out2 : Outport  Port=30
  adc2_data_out3 : Outport  Port=31
  adc2_data_out4 : Outport  Port=32
  adc2_data_out5 : Outport  Port=33
  adc2_data_out6 : Outport  Port=34
  adc2_data_out7 : Outport  Port=35
  adc2_data_out8 : Outport  Port=36
  adc2_data_out9 : Outport  Port=37
  adc3_data_out0 : Outport  Port=38
  adc3_data_out1 : Outport  Port=39
  adc3_data_out2 : Outport  Port=40
  adc3_data_out3 : Outport  Port=41
  adc3_data_out4 : Outport  Port=42
  adc3_data_out5 : Outport  Port=43
  adc3_data_out6 : Outport  Port=44
  adc3_data_out7 : Outport  Port=45
  adc3_data_out8 : Outport  Port=46
  adc3_data_out9 : Outport  Port=47
  wires:
  Slice38/1 -> Reinterpret38/1
  Slice39/1 -> Reinterpret39/1
  Reinterpret38/1 -> adc3_data_out8/1
  Reinterpret39/1 -> adc3_data_out9/1
  Slice37/1 -> Reinterpret29/1
  Slice36/1 -> Reinterpret28/1
  Reinterpret29/1 -> adc2_data_out9/1
  Reinterpret28/1 -> adc2_data_out8/1
  Slice35/1 -> Reinterpret19/1
  Reinterpret19/1 -> adc1_data_out9/1
  Reinterpret18/1 -> adc1_data_out8/1
  Slice34/1 -> Reinterpret18/1
  Reinterpret13/1 -> adc0_data_out9/1
  Reinterpret12/1 -> adc0_data_out8/1
  Slice33/1 -> Reinterpret13/1
  Slice32/1 -> Reinterpret12/1
  xps_library_ADCs_skarab_adc4x3g_14_byp_adc_trigger_out/1 -> adc_trigger_out/1
  Constant10/1 -> xps_library_ADCs_skarab_adc4x3g_14_byp_adc_trigger_out/1
  xps_library_ADCs_skarab_adc4x3g_14_byp_adc_sync_complete_out/1 -> adc_sync_complete_out/1
  Constant9/1 -> xps_library_ADCs_skarab_adc4x3g_14_byp_adc_sync_complete_out/1
  xps_library_ADCs_skarab_adc4x3g_14_byp_pll_sync_complete_out/1 -> pll_sync_complete_out/1
  Constant8/1 -> xps_library_ADCs_skarab_adc4x3g_14_byp_pll_sync_complete_out/1
  Slice29/1 -> Reinterpret37/1
  Reinterpret37/1 -> adc3_data_out7/1
  Slice28/1 -> Reinterpret36/1
  Reinterpret36/1 -> adc3_data_out6/1
  Slice27/1 -> Reinterpret43/1
  Reinterpret43/1 -> adc3_data_out5/1
  Slice26/1 -> Reinterpret42/1
  Reinterpret42/1 -> adc3_data_out4/1
  Slice25/1 -> Reinterpret41/1
  Reinterpret41/1 -> adc3_data_out3/1
  Slice24/1 -> Reinterpret40/1
  Reinterpret40/1 -> adc3_data_out2/1
  Slice31/1 -> Reinterpret35/1
  Reinterpret35/1 -> adc3_data_out1/1
  Slice30/1 -> Reinterpret34/1
  Reinterpret34/1 -> adc3_data_out0/1
  Reinterpret7/1 -> Slice30/1, Slice31/1, Slice24/1, Slice25/1, Slice26/1, Slice27/1, Slice28/1, Slice29/1, Slice38/1, Slice39/1
  xps_library_ADCs_skarab_adc4x3g_14_byp_adc3_data_out/1 -> Reinterpret7/1
  Constant7/1 -> xps_library_ADCs_skarab_adc4x3g_14_byp_adc3_data_out/1
  Slice21/1 -> Reinterpret27/1
  Reinterpret27/1 -> adc2_data_out7/1
  Slice20/1 -> Reinterpret26/1
  Reinterpret26/1 -> adc2_data_out6/1
  Slice19/1 -> Reinterpret33/1
  Reinterpret33/1 -> adc2_data_out5/1
  Slice18/1 -> Reinterpret32/1
  Reinterpret32/1 -> adc2_data_out4/1
  Slice17/1 -> Reinterpret31/1
  Reinterpret31/1 -> adc2_data_out3/1
  Slice16/1 -> Reinterpret30/1
  Reinterpret30/1 -> adc2_data_out2/1
  Slice23/1 -> Reinterpret25/1
  Reinterpret25/1 -> adc2_data_out1/1
  Slice22/1 -> Reinterpret24/1
  Reinterpret24/1 -> adc2_data_out0/1
  Reinterpret5/1 -> Slice22/1, Slice23/1, Slice16/1, Slice17/1, Slice18/1, Slice19/1, Slice20/1, Slice21/1, Slice36/1, Slice37/1
  xps_library_ADCs_skarab_adc4x3g_14_byp_adc2_data_out/1 -> Reinterpret5/1
  Constant3/1 -> xps_library_ADCs_skarab_adc4x3g_14_byp_adc2_data_out/1
  Slice15/1 -> Reinterpret17/1
  Reinterpret17/1 -> adc1_data_out7/1
  Slice14/1 -> Reinterpret16/1
  Reinterpret16/1 -> adc1_data_out6/1
  Slice13/1 -> Reinterpret23/1
  Reinterpret23/1 -> adc1_data_out5/1
  Slice12/1 -> Reinterpret22/1
  Reinterpret22/1 -> adc1_data_out4/1
  Slice11/1 -> Reinterpret21/1
  Reinterpret21/1 -> adc1_data_out3/1
  Slice10/1 -> Reinterpret20/1
  Reinterpret20/1 -> adc1_data_out2/1
  Slice9/1 -> Reinterpret15/1
  Reinterpret15/1 -> adc1_data_out1/1
  Slice8/1 -> Reinterpret14/1
  Reinterpret14/1 -> adc1_data_out0/1
  Reinterpret4/1 -> Slice8/1, Slice9/1, Slice10/1, Slice11/1, Slice12/1, Slice13/1, Slice14/1, Slice15/1, Slice35/1, Slice34/1
  xps_library_ADCs_skarab_adc4x3g_14_byp_adc1_data_out/1 -> Reinterpret4/1
  Constant2/1 -> xps_library_ADCs_skarab_adc4x3g_14_byp_adc1_data_out/1
  Slice7/1 -> Reinterpret11/1
  Reinterpret11/1 -> adc0_data_out7/1
  Slice6/1 -> Reinterpret10/1
  Reinterpret10/1 -> adc0_data_out6/1
  Slice5/1 -> Reinterpret9/1
  Reinterpret9/1 -> adc0_data_out5/1
  Slice4/1 -> Reinterpret8/1
  Reinterpret8/1 -> adc0_data_out4/1
  Slice3/1 -> Reinterpret3/1
  Reinterpret3/1 -> adc0_data_out3/1
  Slice2/1 -> Reinterpret2/1
  Reinterpret2/1 -> adc0_data_out2/1
  Slice1/1 -> Reinterpret1/1
  Reinterpret1/1 -> adc0_data_out1/1
  Slice/1 -> Reinterpret/1
  Reinterpret/1 -> adc0_data_out0/1
  Reinterpret6/1 -> Slice/1, Slice1/1, Slice2/1, Slice3/1, Slice4/1, Slice5/1, Slice6/1, Slice7/1, Slice32/1, Slice33/1
  xps_library_ADCs_skarab_adc4x3g_14_byp_adc0_data_out/1 -> Reinterpret6/1
  Constant6/1 -> xps_library_ADCs_skarab_adc4x3g_14_byp_adc0_data_out/1
  xps_library_ADCs_skarab_adc4x3g_14_byp_adc1_data_val_out/1 -> adc1_data_val_out/1
  Constant5/1 -> xps_library_ADCs_skarab_adc4x3g_14_byp_adc1_data_val_out/1
  xps_library_ADCs_skarab_adc4x3g_14_byp_adc0_data_val_out/1 -> adc0_data_val_out/1
  Constant4/1 -> xps_library_ADCs_skarab_adc4x3g_14_byp_adc0_data_val_out/1
  xps_library_ADCs_skarab_adc4x3g_14_byp_adc3_data_val_out/1 -> adc3_data_val_out/1
  Constant1/1 -> xps_library_ADCs_skarab_adc4x3g_14_byp_adc3_data_val_out/1
  xps_library_ADCs_skarab_adc4x3g_14_byp_adc2_data_val_out/1 -> adc2_data_val_out/1
  Constant/1 -> xps_library_ADCs_skarab_adc4x3g_14_byp_adc2_data_val_out/1
  convert_pll_sync_start_in/1 -> xps_library_ADCs_skarab_adc4x3g_14_byp_pll_sync_start_in/1
  pll_sync_start_in/1 -> convert_pll_sync_start_in/1
  convert_adc_sync_start_in/1 -> xps_library_ADCs_skarab_adc4x3g_14_byp_adc_sync_start_in/1
  adc_sync_start_in/1 -> convert_adc_sync_start_in/1

== system xps_library/ADCs/snap_adc ==
  a1_sim : Inport
  a2_sim : Inport  Port=2
  a3_sim : Inport  Port=3
  a4_sim : Inport  Port=4
  b1_sim : Inport  Port=5
  b2_sim : Inport  Port=6
  b3_sim : Inport  Port=7
  b4_sim : Inport  Port=8
  c1_sim : Inport  Port=9
  c2_sim : Inport  Port=10
  c3_sim : Inport  Port=11
  c4_sim : Inport  Port=12
  xps_library_ADCs_snap_adc_a{1..4} (4 alike) : xbsIndex_r4/Gateway In  gui_display_data_type=Fixed-point  arith_type="Signed  (2's comp)"  n_bits=8  bin_pt=7  preci_type=Single  exp_width=8  frac_width=24  rows=1  columns=1  quantization="Round  (unbiased: +/- Inf)"  overflow=Saturate  period=1  UseAsADC=off  ADCChannel='1'  interface=None  automatic_assignment=on  address_offset=hex2dec('00')  intf_name=''  intf_description=''  default_value=0  timing_constraint=None  locs_specified=off  LOCs={}  io_standard={}  inherit_from_input=off  hdl_port=on  dbl_ovrd=off  block_type=gatewayin
  xps_library_ADCs_snap_adc_b{1..4} (4 alike) : xbsIndex_r4/Gateway In  gui_display_data_type=Fixed-point  arith_type="Signed  (2's comp)"  n_bits=8  bin_pt=7  preci_type=Single  exp_width=8  frac_width=24  rows=1  columns=1  quantization="Round  (unbiased: +/- Inf)"  overflow=Saturate  period=1  UseAsADC=off  ADCChannel='1'  interface=None  automatic_assignment=on  address_offset=hex2dec('00')  intf_name=''  intf_description=''  default_value=0  timing_constraint=None  locs_specified=off  LOCs={}  io_standard={}  inherit_from_input=off  hdl_port=on  dbl_ovrd=off  block_type=gatewayin
  xps_library_ADCs_snap_adc_c{1..4} (4 alike) : xbsIndex_r4/Gateway In  gui_display_data_type=Fixed-point  arith_type="Signed  (2's comp)"  n_bits=8  bin_pt=7  preci_type=Single  exp_width=8  frac_width=24  rows=1  columns=1  quantization="Round  (unbiased: +/- Inf)"  overflow=Saturate  period=1  UseAsADC=off  ADCChannel='1'  interface=None  automatic_assignment=on  address_offset=hex2dec('00')  intf_name=''  intf_description=''  default_value=0  timing_constraint=None  locs_specified=off  LOCs={}  io_standard={}  inherit_from_input=off  hdl_port=on  dbl_ovrd=off  block_type=gatewayin
  a1 : Outport
  a2 : Outport  Port=2
  a3 : Outport  Port=3
  a4 : Outport  Port=4
  b1 : Outport  Port=5
  b2 : Outport  Port=6
  b3 : Outport  Port=7
  b4 : Outport  Port=8
  c1 : Outport  Port=9
  c2 : Outport  Port=10
  c3 : Outport  Port=11
  c4 : Outport  Port=12
  wires:
  a1_sim/1 -> xps_library_ADCs_snap_adc_a1/1
  xps_library_ADCs_snap_adc_a1/1 -> a1/1  "a1"
  a2_sim/1 -> xps_library_ADCs_snap_adc_a2/1
  xps_library_ADCs_snap_adc_a2/1 -> a2/1  "a2"
  a3_sim/1 -> xps_library_ADCs_snap_adc_a3/1
  xps_library_ADCs_snap_adc_a3/1 -> a3/1  "a3"
  a4_sim/1 -> xps_library_ADCs_snap_adc_a4/1
  xps_library_ADCs_snap_adc_a4/1 -> a4/1  "a4"
  b1_sim/1 -> xps_library_ADCs_snap_adc_b1/1
  xps_library_ADCs_snap_adc_b1/1 -> b1/1  "b1"
  b2_sim/1 -> xps_library_ADCs_snap_adc_b2/1
  xps_library_ADCs_snap_adc_b2/1 -> b2/1  "b2"
  b3_sim/1 -> xps_library_ADCs_snap_adc_b3/1
  xps_library_ADCs_snap_adc_b3/1 -> b3/1  "b3"
  b4_sim/1 -> xps_library_ADCs_snap_adc_b4/1
  xps_library_ADCs_snap_adc_b4/1 -> b4/1  "b4"
  c1_sim/1 -> xps_library_ADCs_snap_adc_c1/1
  xps_library_ADCs_snap_adc_c1/1 -> c1/1  "c1"
  c2_sim/1 -> xps_library_ADCs_snap_adc_c2/1
  xps_library_ADCs_snap_adc_c2/1 -> c2/1  "c2"
  c3_sim/1 -> xps_library_ADCs_snap_adc_c3/1
  xps_library_ADCs_snap_adc_c3/1 -> c3/1  "c3"
  c4_sim/1 -> xps_library_ADCs_snap_adc_c4/1
  xps_library_ADCs_snap_adc_c4/1 -> c4/1  "c4"
